simulink model "GainScheduledTest"  (R2020b)
settings: Solver=VariableStepAuto  StartTime=0.0  StopTime=10  RelTol=1e-3
values from neighbouring files (symbols this model uses):
  Inertia = diag([0.0826975856, 0.0826975856, 2.4778e-04])    [StateSpaceController.m]    (also in Tracker.m)
  k_0 = R_uu \ (B' * s_x + r_u)    [Affine_LQR.m]    (also in Trajectory_LQR_fast.m = R_uu \ (B(t)' * s_x + r_u))
  K_x = R_uu \ (B' * S_xx + N')    [Affine_LQR.m]    (also in Trajectory_LQR_fast.m = R_uu \ (B(t)' * S_xx' + N'))
undefined symbols (not defined in the file or in its folder): e0_0, e1_0, e2_0, e3_0
libraries: sharedtransform x3, shared6dofsys x2, sharedutil x1, shared6dof x1
settings Model: Creator=rag  LastModifiedBy=rag
settings OptimizationCC: InitFltsAndDblsToZero=on
settings HardwareCC: ProdLongLongMode=on  TargetLongLongMode=on
settings RTWCC: BuildConfiguration=Faster Runs

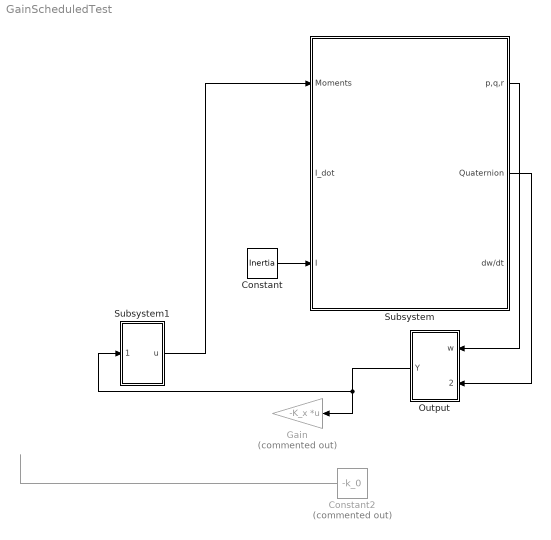
== system GainScheduledTest ==
  Constant : Constant  Value=Inertia
  Constant2 : Constant  Commented=on  Value=-k_0
  Gain : Gain  Commented=on  Gain=-K_x  Multiplication=Matrix(K*u)
  Output : Subsystem
  Subsystem : Subsystem
  Subsystem1 : Subsystem
  wires:
  Output/1(Y) -> Subsystem1/1(state), Gain/1
  Subsystem/2(Quaternion) -> Output/2(error q)
  Subsystem/1(p,q,r) -> Output/1(w)
  Constant/1 -> Subsystem/3(I)
  Constant2/1 -> ?
  Subsystem1/1(u) -> Subsystem/1(Moments)

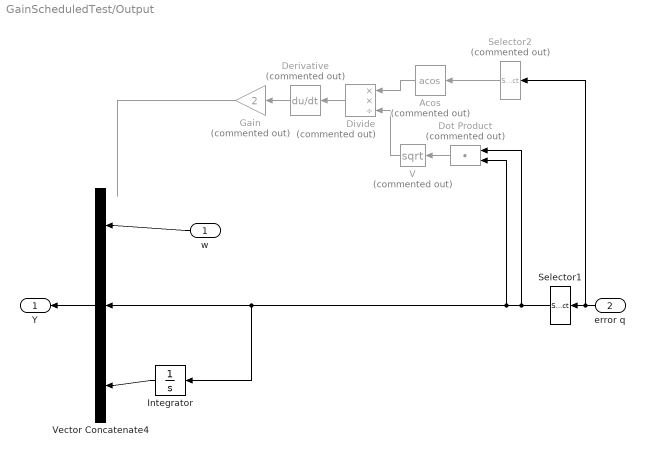
== system GainScheduledTest/Output ==
  w : Inport
  error q : Inport  Port=2
  Acos : Trigonometry  Commented=on  Operator=acos
  Derivative : Derivative  Commented=on
  Divide : Product  Commented=on  Inputs=**/
  Dot Product : DotProduct  Commented=on  SaturateOnIntegerOverflow=on  OutDataTypeStr=Inherit: Inherit via internal rule
  Gain : Gain  Commented=on  Gain=2
  Integrator : Integrator
  Selector1 : Selector  InputPortWidth=4  IndexOptions=Index vector (dialog)  Indices=[2 3 4]  OutputSizes=1
  Selector2 : Selector  Commented=on  InputPortWidth=4  IndexOptions=Index vector (dialog)  Indices=1  OutputSizes=1
  V : Math  Commented=on  Operator=sqrt  SignedPower=on  SaturateOnIntegerOverflow=on
  Vector Concatenate4 : Concatenate  NumInputs=3
  Y : Outport  VectorParamsAs1DForOutWhenUnconnected=off
  wires:
  Vector Concatenate4/1 -> Y/1
  Dot Product/1 -> V/1
  V/1 -> Divide/3
  Acos/1 -> Divide/1
  Selector2/1 -> Acos/1
  Divide/1 -> Derivative/1
  Derivative/1 -> Gain/1
  Gain/1 -> ?
  w/1 -> Vector Concatenate4/1
  error q/1 -> Selector2/1, Selector1/1
  Selector1/1 -> Dot Product/1, Dot Product/2, Integrator/1, Vector Concatenate4/2
  Integrator/1 -> Vector Concatenate4/3

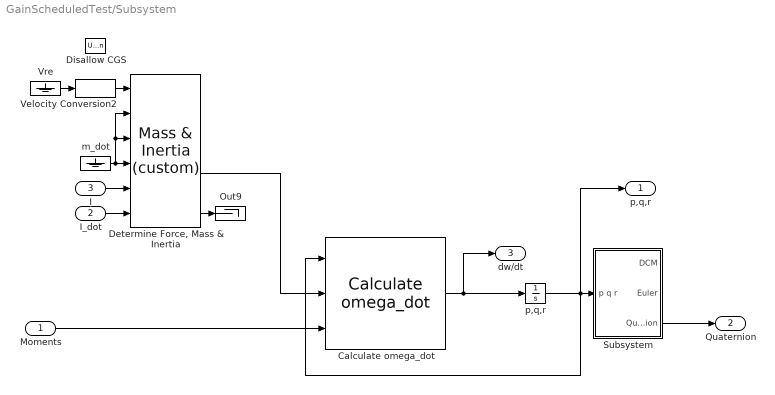
== system GainScheduledTest/Subsystem ==
  Moments : Inport  Unit=N*m  PortDimensions=3
  I_dot : Inport  Port=2  Unit=kg*m^2/s  PortDimensions=[3 3]
  I : Inport  Port=3  Unit=kg*m^2  PortDimensions=[3 3]
  Calculate omega_dot : shared6dofsys/Calculate omega_dot  aMode=aMode
      settings: SourceProductBaseCode=AE,PW,MT,UV,VE,VP
  "Determine Force, Mass & Inertia" : shared6dofsys/Mass & Inertia (custom)  aMode=aMode
      settings: SourceProductBaseCode=AE,PW,MT,UV,VE,VP
  Disallow CGS : UnitConfiguration  UnitSystemsStr=English,SI,SI (extended)  AllowAllUnitSystems=off
  Out9 : Terminator
  Subsystem : Subsystem
  Velocity Conversion2 : shared6dof/6DOF (Euler Angles)/Velocity Conversion2  SystemSampleTime=-1  VariantActivationTime=update diagram  Latency=0  AutoFrameSizeCalculation=off
      settings: SourceProductBaseCode=AE,PW,MT,UV,VE,VP
  Vre : Ground
  m_dot : Ground
  "p,q,r " : Integrator  InitialCondition=[0 0 0]
  p,q,r : Outport  Unit=rad/s  VectorParamsAs1DForOutWhenUnconnected=off
  Quaternion : Outport  Port=2  VectorParamsAs1DForOutWhenUnconnected=off
  dw/dt : Outport  Port=3  VectorParamsAs1DForOutWhenUnconnected=off
  wires:
  "Determine Force, Mass & Inertia"/3 -> Calculate omega_dot/2
  "p,q,r "/1 -> Subsystem/1(p q r), p,q,r/1, Calculate omega_dot/1
  m_dot/1 -> "Determine Force, Mass & Inertia"/2, "Determine Force, Mass & Inertia"/3, "Determine Force, Mass & Inertia"/4
  Calculate omega_dot/1 -> dw/dt/1, "p,q,r "/1
  "Determine Force, Mass & Inertia"/4 -> Out9/1
  I_dot/1 -> "Determine Force, Mass & Inertia"/6
  I/1 -> "Determine Force, Mass & Inertia"/5
  Velocity Conversion2/1 -> "Determine Force, Mass & Inertia"/1
  Vre/1 -> Velocity Conversion2/1
  Subsystem/3(Quaternion) -> Quaternion/1
  Moments/1 -> Calculate omega_dot/3

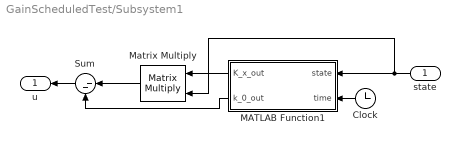
== system GainScheduledTest/Subsystem1 ==
  state : Inport
  Clock : Clock
  MATLAB Function1 : MATLAB Function  TreatAsAtomicUnit=on
  Matrix Multiply : Product  Multiplication=Matrix(*)
  Sum : Sum  Inputs=|--
  u : Outport
  wires:
  Clock/1 -> MATLAB Function1/2(time)
  state/1 -> Matrix Multiply/2, MATLAB Function1/1(state)
  Sum/1 -> u/1
  Matrix Multiply/1 -> Sum/1
  MATLAB Function1/2(k_0_out) -> Sum/2
  MATLAB Function1/1(K_x_out) -> Matrix Multiply/1

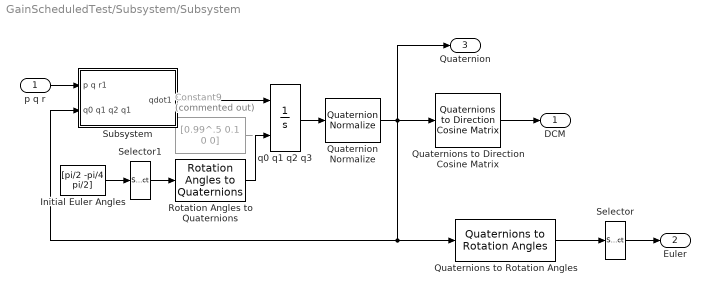
== system GainScheduledTest/Subsystem/Subsystem ==
  p q r : Inport
  Constant9 : Constant  Commented=on  Value=[0.99^.5 0.1 0 0]
  Initial Euler Angles : Constant  Value=[pi/2 -pi/4 pi/2]
  Quaternion Normalize : sharedutil/Quaternion Normalize  aMode=aMode
      settings: SourceProductBaseCode=AE,PW,MT,UV,VE,VP
  Quaternions to Direction Cosine Matrix : sharedtransform/Quaternions to  Direction Cosine Matrix  aMode=aMode
      settings: SourceProductBaseCode=AE,PW,MT,UV,VE,VP
  Quaternions to Rotation Angles : sharedtransform/Quaternions to Rotation Angles  rotationOrder=ZYX  aMode=aMode
      settings: SourceProductBaseCode=AE,PW,MT,UV,VE,VP
  Rotation Angles to Quaternions : sharedtransform/Rotation Angles to Quaternions  rotationOrder=ZYX  aMode=aMode
      settings: SourceProductBaseCode=AE,PW,MT,UV,VE,VP
  Selector : Selector  IndexMode=Zero-based  InputPortWidth=3  IndexOptions=Index vector (dialog)  Indices=[ 2 1 0]  OutputSizes=1
  Selector1 : Selector  IndexMode=Zero-based  InputPortWidth=3  IndexOptions=Index vector (dialog)  Indices=[2 1 0]  OutputSizes=1
  Subsystem : Subsystem
  q0 q1 q2 q3 : Integrator  InitialConditionSource=external  InitialCondition=[e0_0 e1_0 e2_0 e3_0]
  DCM : Outport  VectorParamsAs1DForOutWhenUnconnected=off
  Euler : Outport  Port=2  VectorParamsAs1DForOutWhenUnconnected=off
  Quaternion : Outport  Port=3  VectorParamsAs1DForOutWhenUnconnected=off
  wires:
  Selector/1 -> Euler/1
  Initial Euler Angles/1 -> Selector1/1
  Selector1/1 -> Rotation Angles to Quaternions/1
  q0 q1 q2 q3/1 -> Quaternion Normalize/1
  Quaternions to Direction Cosine Matrix/1 -> DCM/1
  Subsystem/1(qdot1) -> q0 q1 q2 q3/1
  p q r/1 -> Subsystem/1(p q r1)
  Quaternions to Rotation Angles/1 -> Selector/1
  Quaternion Normalize/1 -> Quaternion/1, Subsystem/2(q0 q1 q2 q1), Quaternions to Rotation Angles/1, Quaternions to Direction Cosine Matrix/1
  Rotation Angles to Quaternions/1 -> q0 q1 q2 q3/2
  Constant9/1 -> ?

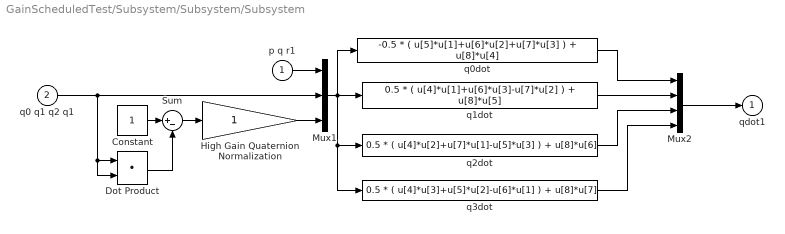
== system GainScheduledTest/Subsystem/Subsystem/Subsystem ==
  p q r1 : Inport
  q0 q1 q2 q1 : Inport  Port=2
  Constant : Constant
  Dot Product : DotProduct  OutDataTypeStr=Inherit: Inherit via internal rule
  High Gain Quaternion Normalization : Gain  SaturateOnIntegerOverflow=on  OutDataTypeStr=Inherit: Same as input  ParamDataTypeStr=Inherit: Same as input
  Mux1 : Mux  Inputs=[3 4 1]
  Mux2 : Mux
  Sum : Sum  Inputs=|+-  InputSameDT=on  SaturateOnIntegerOverflow=on  OutDataTypeStr=Inherit: Same as first input
  q0dot : Fcn  Expr=-0.5 * ( u[5]*u[1]+u[6]*u[2]+u[7]*u[3] ) + u[8]*u[4]
  q1dot : Fcn  Expr=0.5 * ( u[4]*u[1]+u[6]*u[3]-u[7]*u[2] ) + u[8]*u[5]
  q2dot : Fcn  Expr=0.5 * ( u[4]*u[2]+u[7]*u[1]-u[5]*u[3] ) + u[8]*u[6]
  q3dot : Fcn  Expr=0.5 * ( u[4]*u[3]+u[5]*u[2]-u[6]*u[1] ) + u[8]*u[7]
  qdot1 : Outport  InitialOutput=0  VectorParamsAs1DForOutWhenUnconnected=off
  wires:
  Constant/1 -> Sum/1
  Dot Product/1 -> Sum/2
  Mux1/1 -> q2dot/1, q3dot/1, q0dot/1, q1dot/1
  q0 q1 q2 q1/1 -> Dot Product/1, Dot Product/2, Mux1/2
  Sum/1 -> High Gain Quaternion Normalization/1
  Mux2/1 -> qdot1/1
  q0dot/1 -> Mux2/1
  q3dot/1 -> Mux2/4
  q1dot/1 -> Mux2/2
  q2dot/1 -> Mux2/3
  High Gain Quaternion Normalization/1 -> Mux1/3
  p q r1/1 -> Mux1/1

== matlab function GainScheduledTest/Subsystem1/MATLAB Function1 ==
  settings: updateMethod=DISCRETE
  data: state input; K_x_out output; time input; k_0_out output
function [K_x_out, k_0_out] = fcn(state, time)
  coder.extrinsic('affine_controller'); 
  persistent last_time K_x k_0

  if isempty(last_time)
    last_time = 0;
    K_x = zeros(3, 9);
    k_0 = zeros(3, 1);
    [K_x, k_0, ~] = affine_controller(state);
  end
  
  if time - last_time > -1
    [K_x, k_0, ~] = affine_controller(state);
  end
  
  K_x_out = K_x;
  k_0_out = k_0;
  
  last_time = time;
end
